simulink model "sm_motor_grader"  (R2026a)
settings: Solver=daessc  StopTime=stopTime  FixedStep=0.01  AbsTol=1e-3
PostLoadFcn:
  | warning off SimulinkBlock:Foundation:RuntimeAccessInvalidSource
InitFcn:
  | sm_motor_grader_config_initLinkBarHole([bdroot '/Motor Grader'],motGradParams)
StartFcn:
  | tic
StopFcn:
  | Elapsed_Sim_Time = toc;
undefined symbols (not defined in the file): Art, Center, Circle, FL, FR, Grid, LiftL, LiftR, LnL, LnR, Loads, motGradParams, Pin, RFL, RFR, RRL, RRR, Side, StrL, StrR, Tilt, Wheels
libraries: sm_motor_grader_lib x23, sm_lib x11, nesl_utility x10, fl_lib x2, sm_vehicle_utilities_lib x2
(part 1 of 2)
Description:
  | Copyright 2025-2026 The MathWorks, Inc.
settings Model: Creator=gabri  LastModifiedBy=smiller
settings SolverCC: MaxConsecutiveMinStep=5
settings DataIOCC: ExternalInput=activeTestCmds  SignalLoggingName=logsout_sm_motor_grader
settings SimscapeCC: SimscapeNominalValues="[{\"value\":\"1\",\"unit\":\"A\"},{\"value\":\"1\",\"unit\":\"bar\"},{\"value\":\"1\",\"unit\":\"cm^2\"},{\"value\":\"1\",\"unit\":\"cm^3/s\"},{\"value\":\"1\",\"unit\":\"kJ/kg\"},{\"value\":\"1\",\"unit\":\"kW\"},{\"value\":\"1\",\"unit\":\"l\"},{\"value\":\"1\",\"unit\":\"N\"},{\"value\":\"1\",\"unit\":\"N*m\"},{\"value\":\"1\",\"unit\":\"V\"}]"  SimscapeLogName=simlog_sm_motor_grader  SimscapeLogLimitData=off  SimscapeLogDataHistory=5000.0
settings DiagnosticsConfigSet: SimMechanicsConflictingReferenceFrames=none
settings ExplorerConfigSet: InternalSimMechanicsExplorerSettings="<ExplorerConfiguration><canonicalview>default</canonicalview><AnimationSetting><BasePlaybackSpeed>1.0</BasePlaybackSpeed><PlaybackSpeedFactor>2.0</PlaybackSpeedFactor></AnimationSetting><TilePanel><TileInfo><Tiles Columns=\"2\" Count=\"3\" Rows=\"2\"><Column Weight=\"0.5509\"/><Column Weight=\"0.4491\"/><Row Weight=\"0.5\"/><Row Weight=\"0.5\"/><Tile Height=\"1\" Width=\"1\" X=\"0\" Y=\"0\"/><Tile Height=\"1\" Width=\"1\" X=\"0\" Y=\"1\"/><Tile Height=\"2\" Width=\"1\" X=\"1\" Y=\"0\"/></Tiles></TileInfo><SceneInfo><SceneViewer><BGColor><R>1</R><G>1</G><B>1</B></BGColor><Camera><DoPerspective>on</DoPerspective><Position><X>2.67003613633794012</X><Y>-2.42959515750484911e-05</Y><Z>13.0875687442674078</Z></Position><Center><X>2.67003613633794012</X><Y>-2.42959515750484911e-05</Y><Z>12.0875687442674078</Z></Center><Up><X>0</X><Y>1</Y><Z>0</Z></Up><ViewLimDist>1</ViewLimDist><YLim>0.466307658154998583</YLim><XLim>1.14004754858535251</XLim></Camera></SceneViewer><SceneViewer><BGColor><R>1</R><G>1</G><B>1</B></BGColor><Camera><DoPerspective>on</DoPerspective><Position><X>-7.3299638636620621</X><Y>-2.4295951577407715e-05</Y><Z>6.18756874426740744</Z></Position><Center><X>-6.43912840719929225</X><Y>-2.4295951577407715e-05</Y><Z>5.73324266147139472</Z></Center><Up><X>0.454326082796012387</X><Y>-7.7636364860217998e-33</Y><Z>0.890835456462769515</Z></Up><ViewLimDist>1</ViewLimDist><YLim>0.466307658154998583</YLim><XLim>1.14004754858535251</XLim></Camera></SceneViewer><SceneViewer><BGColor><R>1</R><G>1</G><B>1</B></BGColor><Camera><DoPerspective>on</DoPerspective><Position><X>3.08009132544876785</X><Y>3.99997798685902373</Y><Z>0.737659499757807202</Z></Position><Center><X>3.08007769073360693</X><Y>2.99997798720506648</Y><Z>0.737637001317838159</Z></Center><Up><X>-1.85796856891391144e-06</X><Y>-2.24984146382089643e-05</Y><Z>0.999999999745184609</Z></Up><ViewLimDist>1</ViewLimDist><YLim>0.466307658154998583</YLim><XLim>0.457324498365672849</XLim></Camera></SceneViewer></SceneInfo></TilePanel><MechEditorPanel><Cameras><Camera><Id>Camera1</Id><Value><Name>Track FixO FR</Name><NativeCamera><PositionTrackingFeature>Motor_Grader.Vehicle.Camera_Frames.Frame_FixO_FR.R</PositionTrackingFeature><CenterTrackingFeature>Motor_Grader.Vehicle.Camera_Frames.Frame_FixO_FR.R</CenterTrackingFeature><UpVectorTrackingFeature>Motor_Grader.Vehicle.Camera_Frames.Frame_FixO_FR.R</UpVectorTrackingFeature><CenterTrackingOrigin>off</CenterTrackingOrigin><CenterTrackingDirection>+X</CenterTrackingDirection><UpVectorTrackingDirection>+Z</UpVectorTrackingDirection></NativeCamera></Value></Camera><Camera><Id>Camera2</Id><Value><Name>Track FixO Right</Name><NativeCamera><PositionTrackingFeature>Motor_Grader.Vehicle.Camera_Frames.Frame_FixO_Right.R</PositionTrackingFeature><CenterTrackingFeature>Motor_Grader.Vehicle.Camera_Frames.Frame_FixO_Right.R</CenterTrackingFeature><UpVectorTrackingFeature>Motor_Grader.Vehicle.Camera_Frames.Frame_FixO_Right.R</UpVectorTrackingFeature><CenterTrackingOrigin>off</CenterTrackingOrigin><CenterTrackingDirection>+X</CenterTrackingDirection><UpVectorTrackingDirection>+Z</UpVectorTrackingDirection></NativeCamera></Value></Camera><Camera><Id>Camera3</Id><Value><Name>Track FixO RR</Name><NativeCamera><PositionTrackingFeature>Motor_Grader.Vehicle.Camera_Frames.Frame_FixO_RR.R</PositionTrackingFeature><CenterTrackingFeature>Motor_Grader.Vehicle.Camera_Frames.Frame_FixO_RR.R</CenterTrackingFeature><UpVectorTrackingFeature>Motor_Grader.Vehicle.Camera_Frames.Frame_FixO_RR.R</UpVectorTrackingFeature><CenterTrackingOrigin>off</CenterTrackingOrigin><CenterTrackingDirection>+X</CenterTrackingDirection><UpVectorTrackingDirection>+Z</UpVectorTrackingDirection></NativeCamera></Value></Camera><Camera><Id>Camera4</Id><Value><Name>Track FixO RL</Name><NativeCamera><PositionTrackingFeature>Motor_Grader.Vehicle.Camera_Frames.Frame_FixO_RL.R</PositionTrackingFeature><CenterTrackingFeature>Motor_Grader.Vehicle.Camera_Frames.Frame_FixO_RL.R</CenterTrackingFeature><UpVectorTrackingFeature>Motor_Grader.Vehicle.Camera_Frames.Frame_FixO_RL.R</UpVectorTrackingFeature><CenterTrackingOrigin>off</CenterTrackingOrigin><CenterTrackingDirection>+X</CenterTrackingDirection><UpVectorTrackingDirection>+Z</UpVectorTrackingDirection></NativeCamera></Value></Camera><Camera><Id>Camera5</Id><Value><Name>Track FixO Left</Name><NativeCamera><PositionTrackingFeature>Motor_Grader.Vehicle.Camera_Frames.Frame_FixO_Left.R</PositionTrackingFeature><CenterTrackingFeature>Motor_Grader.Vehicle.Camera_Frames.Frame_FixO_Left.R</CenterTrackingFeature><UpVectorTrackingFeature>Motor_Grader.Vehicle.Camera_Frames.Frame_FixO_Left.R</UpVectorTrackingFeature><CenterTrackingOrigin>off</CenterTrackingOrigin><CenterTrackingDirection>+X</CenterTrackingDirection><UpVectorTrackingDirection>+Z</UpVectorTrackingDirection></NativeCamera></Value></Camera><Camera><Id>Camera6</Id><Value><Name>Track FixO FL</Name><NativeCamera><PositionTrackingFeature>Motor_Grader.Vehicle.Camera_Frames.Frame_FixO_FL.R</PositionTrackingFeature><CenterTrackingFeature>Motor_Grader.Vehicle.Camera_Frames.Frame_FixO_FL.R</CenterTrackingFeature><UpVectorTrackingFeature>Motor_Grader.Vehicle.Camera_Frames.Frame_FixO_FL.R</UpVectorTrackingFeature><CenterTrackingOrigin>off</CenterTrackingOrigin><CenterTrackingDirection>+X</CenterTrackingDirection><UpVectorTrackingDirection>+Z</UpVectorTrackingDirection></NativeCamera></Value></Camera><Camera><Id>Camera7</Id><Value><Name>Track FixO Top</Name><NativeCamera><PositionTrackingFeature>Motor_Grader.Vehicle.Camera_Frames.Frame_FixO_Top.R</PositionTrackingFeature><CenterTrackingFeature>Motor_Grader.Vehicle.Camera_Frames.Frame_FixO_Top.R</CenterTrackingFeature><UpVectorTrackingFeature>Motor_Grader.Vehicle.Camera_Frames.Frame_FixO_Top.R</UpVectorTrackingFeature><CenterTrackingOrigin>off</CenterTrackingOrigin><CenterTrackingDirection>+X</CenterTrackingDirection><UpVectorTrackingDirection>+Z</UpVectorTrackingDirection></NativeCamera></Value></Camera><Camera><Id>Camera8</Id><Value><Name>Track FixO Front</Name><NativeCamera><PositionTrackingFeature>Motor_Grader.Vehicle.Camera_Frames.Frame_FixO_Front.R</PositionTrackingFeature><CenterTrackingFeature>Motor_Grader.Vehicle.Camera_Frames.Frame_FixO_Front.R</CenterTrackingFeature><UpVectorTrackingFeature>Motor_Grader.Vehicle.Camera_Frames.Frame_FixO_Front.R</UpVectorTrackingFeature><CenterTrackingOrigin>off</CenterTrackingOrigin><CenterTrackingDirection>+X</CenterTrackingDirection><UpVectorTrackingDirection>+Z</UpVectorTrackingDirection></NativeCamera></Value></Camera><Camera><Id>Camera9</Id><Value><Name>Track FixO Rear</Name><NativeCamera><PositionTrackingFeature>Motor_Grader.Vehicle.Camera_Frames.Frame_FixO_Rear.R</PositionTrackingFeature><CenterTrackingFeature>Motor_Grader.Vehicle.Camera_Frames.Frame_FixO_Rear.R</CenterTrackingFeature><UpVectorTrackingFeature>Motor_Grader.Vehicle.Camera_Frames.Frame_FixO_Rear.R</UpVectorTrackingFeature><CenterTrackingOrigin>off</CenterTrackingOrigin><CenterTrackingDirection>+X</CenterTrackingDirection><UpVectorTrackingDirection>+Z</UpVectorTrackingDirection></NativeCamera></Value></Camera><Camera><Id>Camera10</Id><Value><Name>Track FR</Name><NativeCamera><PositionTrackingFeature>Motor_Grader.Vehicle.Camera_Frames.Frame_FR.R</PositionTrackingFeature><CenterTrackingFeature>Motor_Grader.Vehicle.Camera_Frames.Frame_FR.R</CenterTrackingFeature><UpVectorTrackingFeature>Motor_Grader.Vehicle.Camera_Frames.Frame_FR.R</UpVectorTrackingFeature><CenterTrackingOrigin>off</CenterTrackingOrigin><CenterTrackingDirection>+X</CenterTrackingDirection><UpVectorTrackingDirection>+Z</UpVectorTrackingDirection></NativeCamera></Value></Camera><Camera><Id>Camera11</Id><Value><Name>Track Right</Name><NativeCamera><PositionTrackingFeature>Motor_Grader.Vehicle.Camera_Frames.Frame_Right.R</PositionTrackingFeature><CenterTrackingFeature>Motor_Grader.Vehicle.Camera_Frames.Frame_Right.R</CenterTrackingFeature><UpVectorTrackingFeature>Motor_Grader.Vehicle.Camera_Frames.Frame_Right.R</UpVectorTrackingFeature><CenterTrackingOrigin>off</CenterTrackingOrigin><CenterTrackingDirection>+X</CenterTrackingDirection><UpVectorTrackingDirection>+Z</UpVectorTrackingDirection></NativeCamera></Value></Camera><Camera><Id>Camera12</Id><Value><Name>Track RR</Name><NativeCamera><PositionTrackingFeature>Motor_Grader.Vehicle.Camera_Frames.Frame_RR.R</PositionTrackingFeature><CenterTrackingFeature>Motor_Grader.Vehicle.Camera_Frames.Frame_RR.R</CenterTrackingFeature><UpVectorTrackingFeature>Motor_Grader.Vehicle.Camera_Frames.Frame_RR.R</UpVectorTrackingFeature><CenterTrackingOrigin>off</CenterTrackingOrigin><CenterTrackingDirection>+X</CenterTrackingDirection><UpVectorTrackingDirection>+Z</UpVectorTrackingDirection></NativeCamera></Value></Camera><Camera><Id>Camera13</Id><Value><Name>Track RL</Name><NativeCamera><PositionTrackingFeature>Motor_Grader.Vehicle.Camera_Frames.Frame_RL.R</PositionTrackingFeature><CenterTrackingFeature>Motor_Grader.Vehicle.Camera_Frames.Frame_RL.R</CenterTrackingFeature><UpVectorTrackingFeature>Motor_Grader.Vehicle.Camera_Frames.Frame_RL.R</UpVectorTrackingFeature><CenterTrackingOrigin>off</CenterTrackingOrigin><CenterTrackingDirection>+X</CenterTrackingDirection><UpVectorTrackingDirection>+Z</UpVectorTrackingDirection></NativeCamera></Value></Camera><Camera><Id>Camera14</Id><Value><Name>Track Left</Name><NativeCamera><PositionTrackingFeature>Motor_Grader.Vehicle.Camera_Frames.Frame_Left.R</PositionTrackingFeature><CenterTrackingFeature>Motor_Grader.Vehicle.Camera_Frames.Frame_Left.R</CenterTrackingFeature><UpVectorTrackingFeature>Motor_Grader.Vehicle.Camera_Frames.Frame_Left.R</UpVectorTrackingFeature><CenterTrackingOrigin>off</CenterTrackingOrigin><CenterTrackingDirection>+X</CenterTrackingDirection><UpVectorTrackingDirection>+Z</UpVectorTrackingDirection></NativeCamera></Value></Camera><Camera><Id>Camera15</Id><Value><Name>Track FL</Name><NativeCamera><PositionTrackingFeature>Motor_Grader.Vehicle.Camera_Frames.Frame_FL.R</PositionTrackingFeature><CenterTrackingFeature>Motor_Grader.Vehicle.Camera_Frames.Frame_FL.R</CenterTrackingFeature><UpVectorTrackingFeature>Motor_Grader.Vehicle.Camera_Frames.Frame_FL.R</UpVectorTrackingFeature><CenterTrackingOrigin>off</CenterTrackingOrigin><CenterTrackingDirection>+X</CenterTrackingDirection><UpVectorTrackingDirection>+Z</UpVectorTrackingDirection></NativeCamera></Value></Camera><Camera><Id>Camera16</Id><Value><Name>Track Top</Name><NativeCamera><PositionTrackingFeature>Motor_Grader.Vehicle.Camera_Frames.Frame_Top.R</PositionTrackingFeature><CenterTrackingFeature>Motor_Grader.Vehicle.Camera_Frames.Frame_Top.R</CenterTrackingFeature><UpVectorTrackingFeature>Motor_Grader.Vehicle.Camera_Frames.Frame_Top.R</UpVectorTrackingFeature><CenterTrackingOrigin>off</CenterTrackingOrigin><CenterTrackingDirection>+X</CenterTrackingDirection><UpVectorTrackingDirection>+Z</UpVectorTrackingDirection></NativeCamera></Value></Camera><Camera><Id>Camera17</Id><Value><Name>Track Front</Name><NativeCamera><PositionTrackingFeature>Motor_Grader.Vehicle.Camera_Frames.Frame_Front.R</PositionTrackingFeature><CenterTrackingFeature>Motor_Grader.Vehicle.Camera_Frames.Frame_Front.R</CenterTrackingFeature><UpVectorTrackingFeature>Motor_Grader.Vehicle.Camera_Frames.Frame_Front.R</UpVectorTrackingFeature><CenterTrackingOrigin>off</CenterTrackingOrigin><CenterTrackingDirection>+X</CenterTrackingDirection><UpVectorTrackingDirection>+Z</UpVectorTrackingDirection></NativeCamera></Value></Camera><Camera><Id>Camera18</Id><Value><Name>Track Rear</Name><NativeCamera><PositionTrackingFeature>Motor_Grader.Vehicle.Camera_Frames.Frame_Rear.R</PositionTrackingFeature><CenterTrackingFeature>Motor_Grader.Vehicle.Camera_Frames.Frame_Rear.R</CenterTrackingFeature><UpVectorTrackingFeature>Motor_Grader.Vehicle.Camera_Frames.Frame_Rear.R</UpVectorTrackingFeature><CenterTrackingOrigin>off</CenterTrackingOrigin><CenterTrackingDirection>+X</CenterTrackingDirection><UpVectorTrackingDirection>+Z</UpVectorTrackingDirection></NativeCamera></Value></Camera><Camera><Id>Camera19</Id><Value><Name>Track Blade Front</Name><NativeCamera><PositionTrackingFeature>Motor_Grader.Vehicle.Camera_Frames.Frame_SuspF.R</PositionTrackingFeature><CenterTrackingFeature>Motor_Grader.Vehicle.Camera_Frames.Frame_SuspF.R</CenterTrackingFeature><UpVectorTrackingFeature>Motor_Grader.Vehicle.Camera_Frames.Frame_SuspF.R</UpVectorTrackingFeature><CenterTrackingOrigin>off</CenterTrackingOrigin><CenterTrackingDirection>+X</CenterTrackingDirection><UpVectorTrackingDirection>+Z</UpVectorTrackingDirection></NativeCamera></Value></Camera><Camera><Id>Camera20</Id><Value><Name>Track Blade Rear</Name><NativeCamera><PositionTrackingFeature>Motor_Grader.Vehicle.Camera_Frames.Frame_SuspR.R</PositionTrackingFeature><CenterTrackingFeature>Motor_Grader.Vehicle.Camera_Frames.Frame_SuspR.R</CenterTrackingFeature><UpVectorTrackingFeature>Motor_Grader.Vehicle.Camera_Frames.Frame_SuspR.R</UpVectorTrackingFeature><CenterTrackingOrigin>off</CenterTrackingOrigin><CenterTrackingDirection>+X</CenterTrackingDirection><UpVectorTrackingDirection>+Z</UpVectorTrackingDirection></NativeCamera></Value></Camera><Camera><Id>Camera21</Id><Value><Name>Track Wheel FR</Name><NativeCamera><PositionTrackingFeature>Motor_Grader.Vehicle.Camera_Frames.Frame_Wheel_FR.R</PositionTrackingFeature><CenterTrackingFeature>Motor_Grader.Vehicle.Camera_Frames.Frame_Wheel_FR.R</CenterTrackingFeature><UpVectorTrackingFeature>Motor_Grader.Vehicle.Camera_Frames.Frame_Wheel_FR.R</UpVectorTrackingFeature><CenterTrackingOrigin>off</CenterTrackingOrigin><CenterTrackingDirection>+X</CenterTrackingDirection><UpVectorTrackingDirection>+Z</UpVectorTrackingDirection></NativeCamera></Value></Camera><Camera><Id>Camera22</Id><Value><Name>Track Blade Right</Name><NativeCamera><PositionTrackingFeature>Motor_Grader.Vehicle.Camera_Frames.Frame_Wheel_RR.R</PositionTrackingFeature><CenterTrackingFeature>Motor_Grader.Vehicle.Camera_Frames.Frame_Wheel_RR.R</CenterTrackingFeature><UpVectorTrackingFeature>Motor_Grader.Vehicle.Camera_Frames.Frame_Wheel_RR.R</UpVectorTrackingFeature><CenterTrackingOrigin>off</CenterTrackingOrigin><CenterTrackingDirection>+X</CenterTrackingDirection><UpVectorTrackingDirection>+Z</UpVectorTrackingDirection></NativeCamera></Value></Camera><Camera><Id>Camera23</Id><Value><Name>Track Blade Left</Name><NativeCamera><PositionTrackingFeature>Motor_Grader.Vehicle.Camera_Frames.Frame_Wheel_RL.R</PositionTrackingFeature><CenterTrackingFeature>Motor_Grader.Vehicle.Camera_Frames.Frame_Wheel_RL.R</CenterTrackingFeature><UpVectorTrackingFeature>Motor_Grader.Vehicle.Camera_Frames.Frame_Wheel_RL.R</UpVectorTrackingFeature><CenterTrackingOrigin>off</CenterTrackingOrigin><CenterTrackingDirection>+X</CenterTrackingDirection><UpVectorTrackingDirection>+Z</UpVectorTrackingDirection></NativeCamera></Value></Camera><Camera><Id>Camera24</Id><Value><Name>Track Wheel FL</Name><NativeCamera><PositionTrackingFeature>Motor_Grader.Vehicle.Camera_Frames.Frame_Wheel_FL.R</PositionTrackingFeature><CenterTrackingFeature>Motor_Grader.Vehicle.Camera_Frames.Frame_Wheel_FL.R</CenterTrackingFeature><UpVectorTrackingFeature>Motor_Grader.Vehicle.Camera_Frames.Frame_Wheel_FL.R</UpVectorTrackingFeature><CenterTrackingOrigin>off</CenterTrackingOrigin><CenterTrackingDirection>+X</CenterTrackingDirection><UpVectorTrackingDirection>+Z</UpVectorTrackingDirection></NativeCamera></Value></Camera><Camera><Id>Camera25</Id><Value><Name>View Seat</Name><NativeCamera><PositionTrackingFeature>Motor_Grader.Vehicle.Camera_Frames.Frame_View_Seat_FL.R</PositionTrackingFeature><CenterTrackingFeature>Motor_Grader.Vehicle.Camera_Frames.Frame_View_Seat_FL.R</CenterTrackingFeature><UpVectorTrackingFeature>Motor_Grader.Vehicle.Camera_Frames.Frame_View_Seat_FL.R</UpVectorTrackingFeature><CenterTrackingOrigin>off</CenterTrackingOrigin><CenterTrackingDirection>+X</CenterTrackingDirection><UpVectorTrackingDirection>+Z</UpVectorTrackingDirection></NativeCamera></Value></Camera><Camera><Id>Camera26</Id><Value><Name>View Seat FR</Name><NativeCamera><PositionTrackingFeature>Motor_Grader.Vehicle.Camera_Frames.Frame_View_Seat_FR.R</PositionTrackingFeature><CenterTrackingFeature>Motor_Grader.Vehicle.Camera_Frames.Frame_View_Seat_FR.R</CenterTrackingFeature><UpVectorTrackingFeature>Motor_Grader.Vehicle.Camera_Frames.Frame_View_Seat_FR.R</UpVectorTrackingFeature><CenterTrackingOrigin>off</CenterTrackingOrigin><CenterTrackingDirection>+X</CenterTrackingDirection><UpVectorTrackingDirection>+Z</UpVectorTrackingDirection></NativeCamera></Value></Camera><Camera><Id>Camera27</Id><Value><Name>View Susp FR</Name><NativeCamera><PositionTrackingFeature>Motor_Grader.Vehicle.Camera_Frames.Frame_View_Susp_FR.R</PositionTrackingFeature><CenterTrackingFeature>Motor_Grader.Vehicle.Camera_Frames.Frame_View_Susp_FR.R</CenterTrackingFeature><UpVectorTrackingFeature>Motor_Grader.Vehicle.Camera_Frames.Frame_View_Susp_FR.R</UpVectorTrackingFeature><CenterTrackingOrigin>off</CenterTrackingOrigin><CenterTrackingDirection>+X</CenterTrackingDirection><UpVectorTrackingDirection>+Z</UpVectorTrackingDirection></NativeCamera></Value></Camera><Camera><Id>Camera28</Id><Value><Name>View SaddleR</Name><NativeCamera><PositionTrackingFeature>Motor_Grader.Vehicle.Camera_Frames.Frame_View_Susp_RR.R</PositionTrackingFeature><CenterTrackingFeature>Motor_Grader.Vehicle.Camera_Frames.Frame_View_Susp_RR.R</CenterTrackingFeature><UpVectorTrackingFeature>Motor_Grader.Vehicle.Camera_Frames.Frame_View_Susp_RR.R</UpVectorTrackingFeature><CenterTrackingOrigin>off</CenterTrackingOrigin><CenterTrackingDirection>+X</CenterTrackingDirection><UpVectorTrackingDirection>+Z</UpVectorTrackingDirection></NativeCamera></Value></Camera><Camera><Id>Camera29</Id><Value><Name>View SaddleL</Name><NativeCamera><PositionTrackingFeature>Motor_Grader.Vehicle.Camera_Frames.Frame_View_Susp_RL.R</PositionTrackingFeature><CenterTrackingFeature>Motor_Grader.Vehicle.Camera_Frames.Frame_View_Susp_RL.R</CenterTrackingFeature><UpVectorTrackingFeature>Motor_Grader.Vehicle.Camera_Frames.Frame_View_Susp_RL.R</UpVectorTrackingFeature><CenterTrackingOrigin>off</CenterTrackingOrigin><CenterTrackingDirection>+X</CenterTrackingDirection><UpVectorTrackingDirection>+Z</UpVectorTrackingDirection></NativeCamera></Value></Camera><Camera><Id>Camera30</Id><Value><Name>View Susp FL</Name><NativeCamera><PositionTrackingFeature>Motor_Grader.Vehicle.Camera_Frames.Frame_View_Susp_FL.R</PositionTrackingFeature><CenterTrackingFeature>Motor_Grader.Vehicle.Camera_Frames.Frame_View_Susp_FL.R</CenterTrackingFeature><UpVectorTrackingFeature>Motor_Grader.Vehicle.Camera_Frames.Frame_View_Susp_FL.R</UpVectorTrackingFeature><CenterTrackingOrigin>off</CenterTrackingOrigin><CenterTrackingDirection>+X</CenterTrackingDirection><UpVectorTrackingDirection>+Z</UpVectorTrackingDirection></NativeCamera></Value></Camera><Camera><Id>Camera31</Id><Value><Name>Dolly Camera</Name><NativeCamera><PositionTrackingFeature>Motor_Grader.Vehicle.Camera_Frames.Frame_Dolly.R</PositionTrackingFeature><CenterTrackingFeature>Motor_Grader.Vehicle.Camera_Frames.Frame_Dolly.R</CenterTrackingFeature><UpVectorTrackingFeature>Motor_Grader.Vehicle.Camera_Frames.Frame_Dolly.R</UpVectorTrackingFeature><CenterTrackingOrigin>off</CenterTrackingOrigin><CenterTrackingDirection>+X</CenterTrackingDirection><UpVectorTrackingDirection>+Z</UpVectorTrackingDirection></NativeCamera></Value></Camera><Camera><Id>Camera32</Id><Value><Name>Track Dolly Camera</Name><NativeCamera><PositionTrackingFeature>Motor_Grader.Vehicle.Camera_Frames.Frame_Dolly.R</PositionTrackingFeature><CenterTrackingFeature>Motor_Grader.Vehicle.Camera_Frames.Transform_Camera_Ref.F</CenterTrackingFeature><UpVectorTrackingFeature>Motor_Grader.Vehicle.Camera_Frames.World_Frame.W</UpVectorTrackingFeature><CenterTrackingOrigin>on</CenterTrackingOrigin><UpVectorTrackingDirection>+Z</UpVectorTrackingDirection></NativeCamera></Value></Camera></Cameras><GfxPanelCameraMap><MapElement CameraMLId=\"Camera7\" GfxPanelIndex=\"0\"/><MapElement CameraMLId=\"Camera9\" GfxPanelIndex=\"1\"/><MapElement CameraMLId=\"Camera23\" GfxPanelIndex=\"2\"/></GfxPanelCameraMap><VideoCreator><PlaybackSpeedRatio>1.0</PlaybackSpeedRatio><FrameRate>30</FrameRate><VideoFormat>MPEG-4</VideoFormat><FrameSize>[800 450]</FrameSize></VideoCreator></MechEditorPanel></ExplorerConfiguration>"

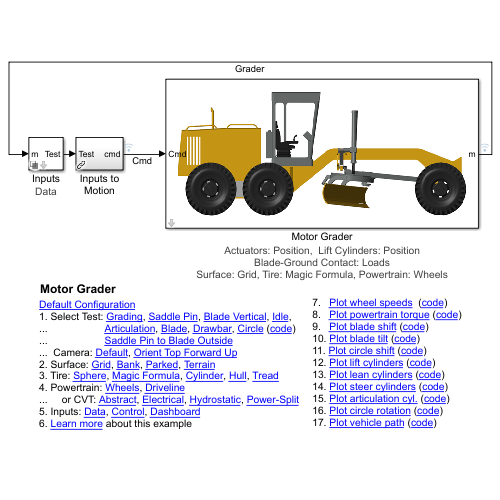
[thumbnail: Simulink's stored preview of the top-level diagram]
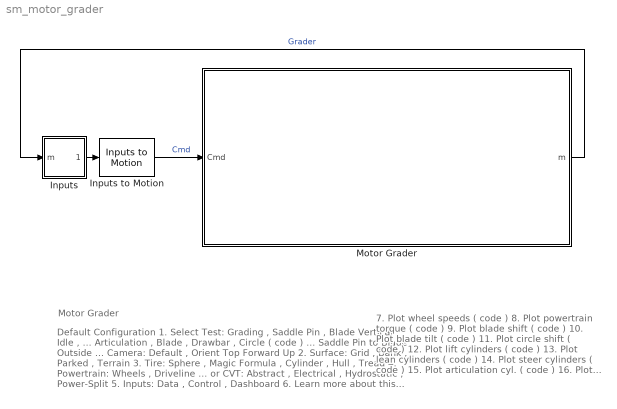
== system sm_motor_grader ==
  note: Default Configuration
      | 1. Select Test: Grading , Saddle Pin , Blade Vertical , Idle ,
      | ... Articulation , Blade , Drawbar , Circle ( code )
      | ... Saddle Pin to Blade Outside
      | ... Camera: Default , Orient Top Forward Up
      | 2. Surface: Grid , Bank , Parked , Terrain
      | 3. Tire: Sphere , Magic Formula , Cylinder , Hull , Tread
      | 4. Powertrain: Wheels , Driveline
      | ... or CVT: Abstract , Electrical , Hydrostatic , Power-Split
      | 5. Inputs: Data , Control , Dashboard
      | 6. Learn more about this example
  note: Motor Grader
  note: 7. Plot wheel speeds ( code )
      | 8. Plot powertrain torque ( code )
      | 9. Plot blade shift ( code )
      | 10. Plot blade tilt ( code )
      | 11. Plot circle shift ( code )
      | 12. Plot lift cylinders ( code )
      | 13. Plot lean cylinders ( code )
      | 14. Plot steer cylinders ( code )
      | 15. Plot articulation cyl. ( code )
      | 16. Plot circle rotation ( code )
      | 17. Plot vehicle path ( code )
  Inputs : Subsystem  Variant=on  VariantControlMode=label  VariantControl=Inputs  LabelModeActiveChoice=Data  mask{test_source=Data}
      mask prompts: test_source "Test Source"
      mask init:
      | bh = gcb;
      | data_source = get_param(bh,'test_source');
      | set_param(bh,'LabelModeActiveChoice',data_source)
      settings: AttributesFormatString=%<LabelModeActiveChoice>
      mask TypeOptions test_source: Data | Dashboard | Control
      mask Display: disp(' ')
  Inputs to Motion : sm_motor_grader_lib/Inputs to Motion  SystemSampleTime=-1  VariantActivationTime=update diagram  EmptyChoice=off  PassThrough=off  PassThroughVariantControl=(default)  EmptyChoiceVariantControl=(default)  AllowFlexibleInterface=on  Latency=0  AutoFrameSizeCalculation=off
  Motor Grader : Subsystem  mask{popup_actuator_model=Position, popup_actuator_model_lift=Position, popup_initial_hole=Center, popup_blade_ground_contact=Loads, popup_ground_contact=Magic Formula, popup_surface_type=Grid, popup_powertrain_config=Wheels}
      mask prompts: popup_actuator_model "Actuation Mode"; popup_actuator_model_lift "Actuation Mode Lift"; popup_initial_hole "Link Bar Initial Hole"; popup_blade_ground_contact "Blade Ground Contact"; popup_ground_contact "Ground Contact"; popup_surface_type "Surface"; popup_powertrain_config "Powertrain Configuration"
      mask init:
      | bh = gcb;
      | modestr = get_param(bh,'popup_actuator_model');
      | set_param([bh '/Vehicle'],'popup_actuator_model',modestr)
      | set_param([bh '/Actuation'],'popup_actuator_model',modestr)
      | 
      | liftmodestr = get_param(bh,'popup_actuator_model_lift');
      | set_param([bh '/Vehicle'],'popup_actuator_model_lift',liftmodestr)
      | set_param([bh '/Actuation'],'popup_actuator_model_lift',liftmodestr)
      settings: AttributesFormatString=|
      | Actuators: %<popup_actuator_model>,  Lift Cylinders: %<popup_actuator_model_lift>
      | Blade-Ground Contact: %<popup_blade_ground_contact>
      | Surface: %<popup_surface_type>, Tire: %<popup_ground_contact>, Powertrain: %<popup_powertrain_config>
      mask TypeOptions popup_actuator_model: Position | Shaft
      mask TypeOptions popup_actuator_model_lift: Position | Shaft
      mask TypeOptions popup_initial_hole: Vehicle/popup_initial_hole
      mask TypeOptions popup_blade_ground_contact: Vehicle/popup_blade_ground_contact
      mask TypeOptions popup_ground_contact: Vehicle/popup_ground_contact
      mask TypeOptions popup_surface_type: Surface/popup_surface_type
      mask TypeOptions popup_powertrain_config: Powertrain/popup_powertrain_config
      mask Display: image('sm_motor_grader_full_IMAGE.png')
  wires:
  Inputs to Motion/1 -> Motor Grader/1(Cmd)  "Cmd"
  Inputs/1(Test) -> Inputs to Motion/1
  Motor Grader/1(m) -> Inputs/1(m)  "Grader"

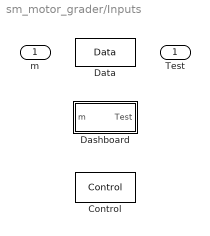
== system sm_motor_grader/Inputs ==
  m : Inport
  Control : sm_motor_grader_lib/Control  SystemSampleTime=-1  VariantControl=Control  VariantActivationTime=update diagram  EmptyChoice=off  PassThrough=off  PassThroughVariantControl=(default)  EmptyChoiceVariantControl=(default)  AllowFlexibleInterface=on  Latency=0  AutoFrameSizeCalculation=off
  Dashboard : Subsystem  VariantControl=Dashboard
  Data : sm_motor_grader_lib/Data  SystemSampleTime=-1  VariantControl=Data  VariantActivationTime=update diagram  EmptyChoice=off  PassThrough=off  PassThroughVariantControl=(default)  EmptyChoiceVariantControl=(default)  AllowFlexibleInterface=on  Latency=0  AutoFrameSizeCalculation=off
  Test : Outport

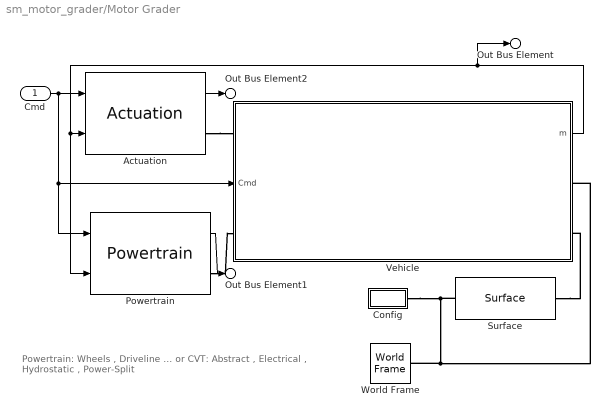
== system sm_motor_grader/Motor Grader ==
  note: Powertrain: Wheels , Driveline
      | ... or CVT: Abstract , Electrical , Hydrostatic , Power-Split
  Cmd : Inport
  Actuation : sm_motor_grader_lib/Actuation  VariantControl=Actuation  popup_actuator_model=Position  popup_actuator_model_lift=Position
  Config : Subsystem
  Powertrain : sm_motor_grader_lib/Powertrain  VariantControl=Powertrain  LabelModeActiveChoice=Torque4  popup_powertrain_config=Wheels
      settings: AttributesFormatString=%<popup_powertrain_config>
  Surface : sm_motor_grader_lib/Surface  VariantControl=Grid  LabelModeActiveChoice=Grid  popup_surface_type=Grid
      settings: AttributesFormatString=%<popup_surface_type>
  Vehicle : Subsystem  mask{popup_actuator_model=Position, popup_actuator_model_lift=Position, popup_initial_hole=Center, popup_ground_contact=Magic Formula, popup_blade_ground_contact=Loads}
      mask prompts: popup_actuator_model "Actuation Mode"; popup_actuator_model_lift "Actuation Mode Lift"; popup_initial_hole "Link Bar Initial Hole"; popup_ground_contact "Ground Contact"; popup_blade_ground_contact "Blade Ground Contact"
      mask init:
      | bh = gcb;
      | modestr = get_param(bh,'popup_actuator_model');
      | set_param([bh '/Frame'],'popup_actuator_model',modestr)
      | set_param([bh '/Frame Front'],'popup_actuator_model',modestr)
      | set_param([bh '/Articulation Cyl'],'popup_actuator_model',modestr)
      | 
      | liftmodestr = get_param(bh,'popup_actuator_model_lift');
      | set_param([bh '/Frame'],'popup_actuator_model_lift',liftmodestr)
      settings: PortSchema="{\"entries\":[{\"content\":{\"sides\":[{\"content\":{\"connectorIds\":[\"LConn1\",\"In1\",\"LConn2\"]},\"type\":\"ConnectorPlacement.EquallySpacedRectSide\",\"uuid\":\"adafa37f-603e-4bbd-8634-b77f5ad2f531\"},{\"content\":{\"connectorIds\":[\"Out1\",\"RConn1\",\"RConn2\"],\"side\":\"RIGHT\"},\"type\":\"ConnectorPlacement.EquallySpacedRectSide\",\"uuid\":\"2f3348e0-ce26-4ee0-aa2b-1c5effb56668\"},{\"content\":{\"side\":\"TOP\"},\"type\":\"ConnectorPlacement.EquallySpacedRectSide\",\"uuid\":\"665560a5-e077-4854-b4fb-3e40ee17391f\"}]},\"type\":\"ConnectorPlacement.EquallySpacedConnector\",\"uuid\":\"512ced80-fdc2-44af-923d-49b4b897b3c0\"}],\"packageUris\":[\"http://schema.mathworks.com/mf0/Connector/R2020b\"],\"version\":\"1.0\"}"
      mask TypeOptions popup_actuator_model: Position | Shaft
      mask TypeOptions popup_actuator_model_lift: Position | Shaft
      mask TypeOptions popup_initial_hole: Frame/popup_initial_hole
      mask TypeOptions popup_ground_contact: Frame Rear/popup_ground_contact | Frame Front/popup_ground_contact
      mask TypeOptions popup_blade_ground_contact: Frame/popup_blade_ground_contact
      mask Display: image('sm_motor_grader_full_IMAGE.png')
  World Frame : sm_lib/Frames and Transforms/World Frame
  Out Bus Element : Outport  PortName=m  Element=Vehicle
  Out Bus Element1 : Outport  PortName=m  Element=Powertrain
  Out Bus Element2 : Outport  PortName=m  Element=Actuation
  wires:
  Cmd/1 -> Actuation/1, Vehicle/1(Cmd), Powertrain/1
  Vehicle/1(m) -> Out Bus Element/1, Powertrain/2, Actuation/2
  Powertrain/1 -> Out Bus Element1/1
  Actuation/1 -> Out Bus Element2/1
  connections:
  Powertrain/RConn1 -- Vehicle/LConn2
  Actuation/RConn1 -- Vehicle/LConn1
  Surface/LConn1 -- Config/RConn1 -- Vehicle/RConn1 -- World Frame/RConn1
  Surface/RConn1 -- Vehicle/RConn2

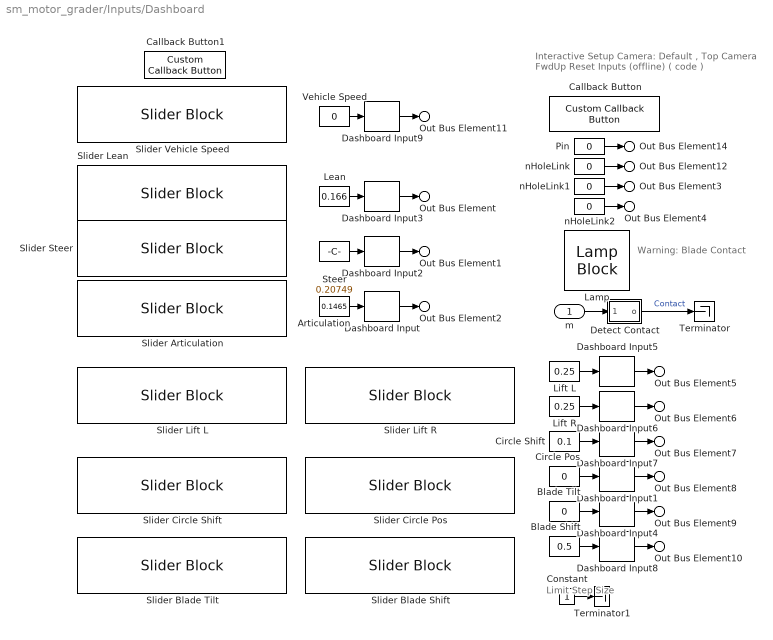
== system sm_motor_grader/Inputs/Dashboard ==
  note: Warning:
      | Blade Contact
  note: Interactive Setup
      | Camera: Default , Top Camera FwdUp
      | Reset Inputs (offline) ( code )
  note: Limit Step Size
  m : Inport
  Articulation : Constant  Value=0.1465
  Blade Shift : Constant  Value=0.5
  Blade Tilt : Constant  Value=0
  Callback Button : CustomCallbackButton  Configuration="{\"components\":[{\"name\":\"BackgroundImageComponent\",\"settings\":{\"image\":{\"size\":[0,0],\"src\":\"default\",\"srcOrientation\":\"Right\"},\"position\":[0,0,1,1]}},{\"name\":\"ButtonStateComponent\",\"settings\":{\"buttonType\":\"momentary\",\"clickFcn\":\"sm_motor_grader_init_dashboard_values(gcs,motGradParams)\",\"onValue\":1,\"position\":[0,0,1,1],\"pressDelay\":\"500\",\"pressFcn\":\"\",\"repeatInterval\":\"0\",\"states\":[{\"horizontalAlignment\":\"center\",\"image\":{\"position\":[0,0,1,1],\"size\":[1,1],\"src\":\"default\",\"srcOrientation\":\"Right\"},\"label\":{\"color\":[0.01176470588,0.01176470588,0.01176470588,1],\"icon\":{\"size\":[0,0],\"src\":\"default\",\"srcOrientation\":\"Right\"},\"iconOffset\":0,\"iconPlacement\":\"left\",\"opacity\":1,\"show\":true,\"text\":{\"content\":\"Reset Inputs\",\"font\":\"Arial\"}},\"labelOffset\":[0,0],\"verticalAlignment\":\"middle\"},{\"horizontalAlignment\":\"center\",\"image\":{\"position\":[0,0,1,1],\"size\":[1,1],\"src\":\"default\",\"srcOrientation\":\"Right\"},\"label\":{\"color\":[0.01176470588,0.01176470588,0.01176470588,1],\"icon\":{\"size\":[0,0],\"src\":\"default\",\"srcOrientation\":\"Right\"},\"iconOffset\":0,\"iconPlacement\":\"left\",\"opacity\":1,\"show\":true,\"text\":{\"content\":\"Reset Inputs\",\"font\":\"Arial\"}},\"labelOffset\":[0,0],\"verticalAlignment\":\"middle\"},{\"horizontalAlignment\":\"center\",\"image\":{\"position\":[0,0,1,1],\"size\":[1,1],\"src\":\"default\",\"srcOrientation\":\"Right\"},\"label\":{\"color\":[0.01176470588,0.01176470588,0.01176470588,1],\"icon\":{\"size\":[0,0],\"src\":\"default\",\"srcOrientation\":\"Right\"},\"iconOffset\":0,\"iconPlacement\":\"left\",\"opacity\":1,\"show\":true,\"text\":{\"content\":\"Reset Inputs\",\"font\":\"Arial\"}},\"labelOffset\":[0,0],\"verticalAlignment\":\"middle\"},{\"horizontalAlignment\":\"center\",\"image\":{\"position\":[0,0,1,1],\"size\":[1,1],\"src\":\"default\",\"srcOrientation\":\"Right\"},\"label\":{\"color\":[0.01176470588,0.01176470588,0.01176470588,1],\"icon\":{\"size\":[0,0],\"src\":\"default\",\"srcOrientation\":\"Right\"},\"iconOffset\":0,\"iconPlacement\":\"left\",\"opacity\":1,\"show\":true,\"text\":{\"content\":\"Reset Inputs\",\"font\":\"Arial\"}},\"labelOffset\":[0,0],\"verticalAlignment\":\"middle\"}]}},{\"name\":\"ForegroundImageComponent\",\"settings\":{\"image\":{\"size\":[0,0],\"src\":\"default\",\"srcOrientation\":\"Right\"},\"isForeground\":1,\"position\":[0,0,1,1]}}],\"settings\":{\"BindingType\":\"standalone\",\"backgroundColor\":[244,244,244,1],\"backgroundOffset\":0.2,\"backgroundOpacity\":1,\"fixedAspectRatio\":\"off\",\"foregroundColor\":[0.01176470588,0.01176470588,0.01176470588,1],\"migratedFromLegacy\":true,\"useBackgroundColor\":true,\"variant\":\"callback\",\"version\":\"R2023a\"},\"type\":\"Button\"}"  CustomBackgroundColor="{\"color\":[0.9568627451,0.9568627451,0.9568627451],\"show\":true}"
  Callback Button1 : CustomCallbackButton  Configuration="{\"components\":[{\"name\":\"BackgroundImageComponent\",\"settings\":{\"image\":{\"size\":[0,0],\"src\":\"default\",\"srcOrientation\":\"Right\"},\"position\":[0,0,1,1]}},{\"name\":\"ButtonStateComponent\",\"settings\":{\"buttonType\":\"momentary\",\"clickFcn\":\"set_param([gcs '\\/Vehicle Speed'],'Value','0')\",\"onValue\":1,\"position\":[0,0,1,1],\"pressDelay\":\"500\",\"pressFcn\":\"\",\"repeatInterval\":\"0\",\"states\":[{\"horizontalAlignment\":\"center\",\"image\":{\"position\":[0,0,1,1],\"size\":[1,1],\"src\":\"default\",\"srcOrientation\":\"Right\"},\"label\":{\"color\":[0.01176470588,0.01176470588,0.01176470588,1],\"icon\":{\"size\":[0,0],\"src\":\"default\",\"srcOrientation\":\"Right\"},\"iconOffset\":0,\"iconPlacement\":\"left\",\"opacity\":1,\"show\":true,\"text\":{\"content\":\"Stop Grader\",\"font\":\"Arial\"}},\"labelOffset\":[0,0],\"verticalAlignment\":\"middle\"},{\"horizontalAlignment\":\"center\",\"image\":{\"position\":[0,0,1,1],\"size\":[1,1],\"src\":\"default\",\"srcOrientation\":\"Right\"},\"label\":{\"color\":[0.01176470588,0.01176470588,0.01176470588,1],\"icon\":{\"size\":[0,0],\"src\":\"default\",\"srcOrientation\":\"Right\"},\"iconOffset\":0,\"iconPlacement\":\"left\",\"opacity\":1,\"show\":true,\"text\":{\"content\":\"Stop Grader\",\"font\":\"Arial\"}},\"labelOffset\":[0,0],\"verticalAlignment\":\"middle\"},{\"horizontalAlignment\":\"center\",\"image\":{\"position\":[0,0,1,1],\"size\":[1,1],\"src\":\"default\",\"srcOrientation\":\"Right\"},\"label\":{\"color\":[0.01176470588,0.01176470588,0.01176470588,1],\"icon\":{\"size\":[0,0],\"src\":\"default\",\"srcOrientation\":\"Right\"},\"iconOffset\":0,\"iconPlacement\":\"left\",\"opacity\":1,\"show\":true,\"text\":{\"content\":\"Stop Grader\",\"font\":\"Arial\"}},\"labelOffset\":[0,0],\"verticalAlignment\":\"middle\"},{\"horizontalAlignment\":\"center\",\"image\":{\"position\":[0,0,1,1],\"size\":[1,1],\"src\":\"default\",\"srcOrientation\":\"Right\"},\"label\":{\"color\":[0.01176470588,0.01176470588,0.01176470588,1],\"icon\":{\"size\":[0,0],\"src\":\"default\",\"srcOrientation\":\"Right\"},\"iconOffset\":0,\"iconPlacement\":\"left\",\"opacity\":1,\"show\":true,\"text\":{\"content\":\"Stop Grader\",\"font\":\"Arial\"}},\"labelOffset\":[0,0],\"verticalAlignment\":\"middle\"}]}},{\"name\":\"ForegroundImageComponent\",\"settings\":{\"image\":{\"size\":[0,0],\"src\":\"default\",\"srcOrientation\":\"Right\"},\"isForeground\":1,\"position\":[0,0,1,1]}}],\"settings\":{\"BindingType\":\"standalone\",\"backgroundColor\":[244,244,244,1],\"backgroundOffset\":0.2,\"backgroundOpacity\":1,\"fixedAspectRatio\":\"off\",\"foregroundColor\":[0.01176470588,0.01176470588,0.01176470588,1],\"migratedFromLegacy\":true,\"useBackgroundColor\":true,\"variant\":\"callback\",\"version\":\"R2023a\"},\"type\":\"Button\"}"  CustomBackgroundColor="{\"color\":[0.9568627451,0.9568627451,0.9568627451],\"show\":true}"
  Circle Pos : Constant  Value=0
  Circle Shift : Constant  Value=0.1
  Constant : Constant  SampleTime=0.05
  Dashboard Input : sm_motor_grader_lib/Dashboard Input  upper_bound=motGradParams.articulation.upperBound  lower_bound=motGradParams.articulation.lowerBound  U0=motGradParams.articulation.initPos  tfilt=1
  Dashboard Input1 : sm_motor_grader_lib/Dashboard Input  upper_bound=motGradParams.circleRot.maxPos  lower_bound=motGradParams.circleRot.minPos  U0=motGradParams.circleRot.initPos  tfilt=1
  Dashboard Input2 : sm_motor_grader_lib/Dashboard Input  upper_bound=motGradParams.steer.upperBound  lower_bound=motGradParams.steer.lowerBound  U0=motGradParams.steer.initPos  tfilt=1
  Dashboard Input3 : sm_motor_grader_lib/Dashboard Input  upper_bound=motGradParams.wheelLean.upperBound  lower_bound=motGradParams.wheelLean.lowerBound  U0=motGradParams.wheelLean.initPos  tfilt=1
  Dashboard Input4 : sm_motor_grader_lib/Dashboard Input  upper_bound=motGradParams.bladeTilt.stroke  lower_bound=0  U0=motGradParams.bladeTilt.initPos  tfilt=0.1
  Dashboard Input5 : sm_motor_grader_lib/Dashboard Input  upper_bound=motGradParams.bladeLift.stroke  lower_bound=0  U0=motGradParams.bladeLift.leftInitPos  tfilt=0.1
  Dashboard Input6 : sm_motor_grader_lib/Dashboard Input  upper_bound=motGradParams.bladeLift.stroke  lower_bound=0  U0=motGradParams.bladeLift.rightInitPos  tfilt=0.1
  Dashboard Input7 : sm_motor_grader_lib/Dashboard Input  upper_bound=motGradParams.circleShift.stroke  lower_bound=0  U0=motGradParams.circleShift.initPos  tfilt=0.1
  Dashboard Input8 : sm_motor_grader_lib/Dashboard Input  upper_bound=motGradParams.bladeSideShift.stroke  lower_bound=0  U0=motGradParams.bladeSideShift.initPos  tfilt=0.1
  Dashboard Input9 : sm_motor_grader_lib/Dashboard Input  upper_bound=motGradParams.drivetrain.topSpeed  lower_bound=-motGradParams.drivetrain.topSpeed  U0=0  tfilt=1
  Detect Contact : Subsystem
  Lamp : LampBlock  LabelPosition=Hide  DefaultColor=[192.0, 192.0, 192.0]
  Lean : Constant  Value=0.166
  Lift L : Constant  Value=0.25
  Lift R : Constant  Value=0.25
  Pin : Constant  Value=0
  Slider Articulation : SliderBlock  ScaleMin=0.076499999999999985  ScaleMax=0.2165
  Slider Blade Shift : SliderBlock  ScaleMax=1.3
  Slider Blade Tilt : SliderBlock  ScaleMax=0.20000000000000001
  Slider Circle Pos : SliderBlock  ScaleMin=-90  ScaleMax=90
  Slider Circle Shift : SliderBlock  ScaleMax=0.84999999999999998
  Slider Lean : SliderBlock  ScaleMin=0.10000000000000001  ScaleMax=0.23200000000000001
  Slider Lift L : SliderBlock  ScaleMax=1.2
  Slider Lift R : SliderBlock  ScaleMax=1.2
  Slider Steer : SliderBlock  ScaleMin=0.14748700000000001  ScaleMax=0.26748700000000003
  Slider Vehicle Speed : SliderBlock  ScaleMin=-11  ScaleMax=11
  Steer : Constant  Value=0.20749
  Terminator : Terminator
  Terminator1 : Terminator
  Vehicle Speed : Constant  Value=0
  nHoleLink : Constant  Value=0
  nHoleLink1 : Constant  Value=0
  nHoleLink2 : Constant  Value=0
  Out Bus Element : Outport  PortName=Test  Element=pLean
  Out Bus Element1 : Outport  PortName=Test  Element=pSteer
  Out Bus Element2 : Outport  PortName=Test  Element=pArtic
  Out Bus Element5 : Outport  PortName=Test  Element=pLiftL
  Out Bus Element6 : Outport  PortName=Test  Element=pLiftR
  Out Bus Element7 : Outport  PortName=Test  Element=pCircleShift
  Out Bus Element8 : Outport  PortName=Test  Element=qCircle
  Out Bus Element9 : Outport  PortName=Test  Element=pTilt
  Out Bus Element10 : Outport  PortName=Test  Element=pShift
  Out Bus Element11 : Outport  PortName=Test  Element=vVeh
  Out Bus Element12 : Outport  PortName=Test  Element=nHoleLink
  Out Bus Element14 : Outport  PortName=Test  Element=pPin
  Out Bus Element3 : Outport  PortName=Test  Element=mLiftL
  Out Bus Element4 : Outport  PortName=Test  Element=mLiftR
  wires:
  Dashboard Input9/1 -> Out Bus Element11/1
  Vehicle Speed/1 -> Dashboard Input9/1
  Lift L/1 -> Dashboard Input5/1
  Lift R/1 -> Dashboard Input6/1
  Circle Shift/1 -> Dashboard Input7/1
  Circle Pos/1 -> Dashboard Input1/1
  Blade Tilt/1 -> Dashboard Input4/1
  Blade Shift/1 -> Dashboard Input8/1
  Lean/1 -> Dashboard Input3/1
  Steer/1 -> Dashboard Input2/1
  Dashboard Input/1 -> Out Bus Element2/1
  nHoleLink/1 -> Out Bus Element12/1
  Pin/1 -> Out Bus Element14/1
  Articulation/1 -> Dashboard Input/1
  Dashboard Input1/1 -> Out Bus Element8/1
  Dashboard Input2/1 -> Out Bus Element1/1
  Dashboard Input3/1 -> Out Bus Element/1
  Dashboard Input4/1 -> Out Bus Element9/1
  Dashboard Input5/1 -> Out Bus Element5/1
  Dashboard Input6/1 -> Out Bus Element6/1
  Dashboard Input7/1 -> Out Bus Element7/1
  Dashboard Input8/1 -> Out Bus Element10/1
  m/1 -> Detect Contact/1(m)
  Detect Contact/1(o) -> Terminator/1  "Contact"
  nHoleLink1/1 -> Out Bus Element3/1
  nHoleLink2/1 -> Out Bus Element4/1
  Constant/1 -> Terminator1/1

== system sm_motor_grader/Motor Grader/Config ==
  Mechanism Configuration : sm_lib/Utilities/Mechanism Configuration  UniformGravity=Constant  GravityVector=[0 0 -9.80665]  GravityVectorUnits=m/s^2  LinearizationDelta=0.001  JointModeTransitionNonlinearIterations=2
  Solver Configuration : nesl_utility/Solver Configuration  PhysicalDomain=network_engine_domain  SubClassName=solver  LeftPortType=input  RightPortType=generic  Tones=[]  Harmonics=[]  SimulateNoise=off  Profile=off  UseLocalSampling=off  EnableSwitchedLinearOptims=on  FrequencyDomain=off  UseCCode=off  RelTol=0.001  AbsTol=0.001  MinStep=1e-09  ToWorkspace=off  RevertToSquareIcSolve=off  NumHomotopyIterations=100  PhasorMode=off  PhasorModeNumHarmonics=1  ConsistencySolver=NEWTON_XTOL_AFTER_FTOL  CanonicalOrdering=UNORDERED  OptimizeIntermediates=UNOPTIMIZED  IndexReductionMethod=DerivativeReplacement  DoDC=off  ResidualTolerance=1e-09  ConsistencyTolSource=GLOBAL  ConsistencyAbsTol=0.001  ConsistencyRelTol=0.001  ConsistencyTolFactor=0.001  UseLocalSolver=off  LocalSolverChoice=NE_BACKWARD_EULER_ADVANCER  ResolveIndetEquations=on  FunctionEvalNumThread=1  LocalSolverSampleTime=0.001  DoFixedCost=off  MaxNonlinIter=3  MaxModeIter=2  ComputeImpulses=off  ImpulseIterations=2  LinearAlgebra=auto  LinearAlgebraNumThread=0  EquationFormulation=NE_TIME_EF  DelaysMemoryBudget=1024  AutomaticFiltering=on  FilteringTimeConstant=0.001  PartitionStorageMethod=AS_NEEDED  PartitionMemoryBudget=1024  PartitionMethod=ROBUST  MultibodyUseLocalSolver=off  MultibodyLocalSolverChoice=ODE1  MultibodyLocalSolverSampleTime=0.001
  W : PMIOPort  Side=Right
  connections:
  Solver Configuration/RConn1 -- W/RConn1 -- Mechanism Configuration/RConn1
